simulink model "ExampleDifferential"  (Simulink 9.2)
settings: Solver=FixedStepDiscrete  StartTime=0.0  StopTime=10.0  FixedStep=" 0.0025"  RelTol=1e-3  EnableMultiTasking=on
libraries: rFproPhysicsLib x4
Description:
  | Compiled Plugin Only
settings Model: Creator=enewton  LastModifiedBy=SeanKavanagh
settings OptimizationCC: ExpressionDepthLimit=2147483647
settings DebuggingCC: SolverPrmCheckMsg=warning  InheritedTsInSrcMsg=none
settings RTWCC: SystemTargetFile=rfpro.tlc  MakeCommand="make_rtw OPTS=\"-DCOMPUTE_DIFF\""  TemplateMakefile=rfpro.tmf  Description=r-Factor Pro Target (Compute Diff Transfer)  TargetLang=C++
settings STFCustomTargetCC: ModelReferenceCompliant=off  GeneratePreprocessorConditionals=Disable all  CombineOutputUpdateFcns=on  MatFileLogging=on  CPPClassGenCompliant=on  GRTInterface=off  SystemTargetFile=rfpro.tlc
settings GRTTargetCC: ModelReferenceCompliant=off  ParMdlRefBuildCompliant=off  CompOptLevelCompliant=off  ConcurrentExecutionCompliant=off  CombineOutputUpdateFcns=on  GRTInterface=off  UseToolchainInfoCompliant=off  ExtModeMexFile=noextcomm

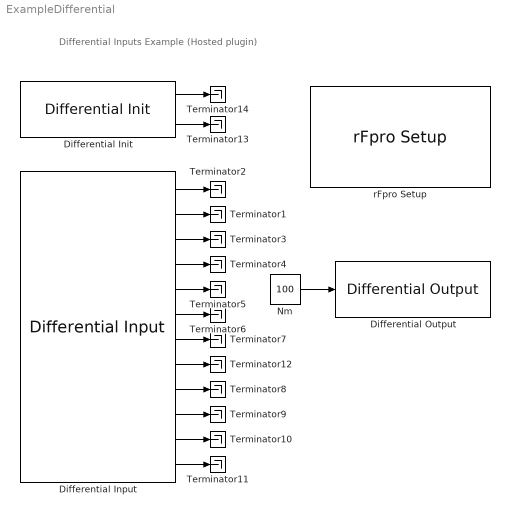
== system ExampleDifferential ==
  note: Differential Inputs Example (Hosted plugin)
  Differential Init : rFproPhysicsLib/Hosted Blocks/Differential Init  SFunctionModules=''
  Differential Input : rFproPhysicsLib/Hosted Blocks/Differential Input  SFunctionModules=''
  Differential Output : rFproPhysicsLib/Hosted Blocks/Differential Output  SFunctionModules=''
  Nm : Constant  Value=100
  Terminator{1..14} (14 alike) : Terminator
  rFpro Setup : rFproPhysicsLib/rFpro Setup  Priority=1  platform=Hosted Plugin  stopOnSessionEnd=on  usePseudoRealtime=on  syncToRF=on  useReverseByteOrder=off  useRfTime=on  minIterations=4  maxIterations=1000  ipReceiveAddress='127.0.0.1'  ipReceivePort=11054  receiveSampleTime=-1  ipTransmitAddress='127.0.0.1'  ipTransmitPort=11052  transmitSampleTime=-1  pluginType=COMPUTE_DIFF
  wires:
  Differential Input/1 -> Terminator2/1
  Differential Input/2 -> Terminator1/1
  Differential Input/3 -> Terminator3/1
  Differential Input/4 -> Terminator4/1
  Differential Input/5 -> Terminator5/1
  Differential Input/6 -> Terminator6/1
  Differential Input/7 -> Terminator7/1
  Differential Input/9 -> Terminator8/1
  Differential Input/10 -> Terminator9/1
  Differential Input/11 -> Terminator10/1
  Differential Input/12 -> Terminator11/1
  Differential Input/8 -> Terminator12/1
  Nm/1 -> Differential Output/1
  Differential Init/1 -> Terminator14/1
  Differential Init/2 -> Terminator13/1
